simulink model "QuadcopterSimModel_INDI_Traj"  (R2018b)
settings: Solver=ode23  StartTime=0.0  StopTime=1000  FixedStep=sample_time  RelTol=1e-4  EnableMultiTasking=on
undefined symbols (not defined in the file): alt_ground, atmosphere, cycle, DiscIntNeverNeededParam, envir, fm_loiter, g, jystck, pos_ref, sigbuilder_block, traj_empty, waypoints, wind
libraries: simulink x6, ndi_lib x5, filters_lib x5, axes_transformation_lib x4, angles_lib x3, unit_conversions_lib x3, cntrl_atti_red_indi_lib x2, traj_lib x2, aerolibfltsims x2, control_allocation_lib x1, sensors_lib x1, atmosphere_lib x1
(part 3 of 3)

== matlab function QuadcopterSimModel_INDI_Traj/Controller INDI/Multicopter INDI Loiter Flight Mode/Multicopter Altitude Hold Flight Mode with INDI and reduced attitude control/control effectiveness/MATLAB Function ==
  data: ny_du_red_trim input; ny_du_dt_trim input; u_trim input; u input; G1 output; T_s input; G2 output
function [G1,G2] = controlEffectiveness2G1G2( ny_du_red_trim, ny_du_dt_trim, u_trim, u, T_s) %#codegen
[G1,G2] = controlEffectiveness2G1G2( ny_du_red_trim, ny_du_dt_trim, u_trim, u, T_s);
end

== matlab function QuadcopterSimModel_INDI_Traj/Controller INDI/Multicopter INDI Loiter Flight Mode/Multicopter Altitude Hold Flight Mode with INDI and reduced attitude control/Multicopter (Reduced) Attitude INDI Controller/reference model/MATLAB Function ==
  data: n_b_d output; n_b_d_dt output; omega_Kb input; n_b_d_dt2 output; omega_Kb_dt input; M_bg input; n_g_d input; n_g_d_dt input; n_g_d_dt2 input
function [ n_b_d, n_b_d_dt, n_b_d_dt2]   = fcn(omega_Kb, omega_Kb_dt, M_bg, n_g_d, n_g_d_dt, n_g_d_dt2 )
% https://arxiv.org/pdf/2002.07837.pdf

% time derivative of rotation matrix
M_bg_dt = dcmDerivFromOmega( M_bg', omega_Kb )';

n_b_d = M_bg*n_g_d;

n_b = single([0;0;-1]);
rho = acos( max( -1, min( 1, dot( n_b_d, n_b ) ) ) );

% eq. (7)
n_b_d_dt = -cross(omega_Kb,n_b_d) + M_bg*n_g_d_dt;

% time derivative of eq. (7)
n_b_d_dt2 = -cross(omega_Kb_dt,n_b_d) -cross(omega_Kb,n_b_d_dt) ...
    + M_bg_dt*n_g_d_dt + M_bg*n_g_d_dt2;

% manipulate desired vector if it is tilted more than 90 degrees
if n_b_d(3) > 0
    n_b_d(3) = 0;
    %n_b_d = n_b_d/(eps(n_b_d(1))+norm(n_b_d,2));
    % increase h1 and h2 up to 2 (2 for 180 degrees)
    n_b_d(1:2) = n_b_d(1:2) + 2*( n_b_d(1:2)/(eps(n_b_d(1))+norm(n_b_d(1:2),2)) - n_b_d(1:2) );
    if norm(n_b_d,2) < 0.9
        n_b_d(1) = -1;
        n_b_d = n_b_d/norm(n_b_d,2);
    end
    % sign must be flipped but it yields better results if the magnitude is
    % reduced
    n_b_d_dt = -n_b_d_dt*0.2;
    n_b_d_dt2 = -n_b_d_dt2*0.2;
end

end

== matlab function QuadcopterSimModel_INDI_Traj/Controller INDI/Multicopter INDI Loiter Flight Mode/Multicopter Altitude Hold Flight Mode with INDI and reduced attitude control/Multicopter (Reduced) Attitude INDI Controller/reference model/MATLAB Function1 ==
  data: n_b_d output; n_b_d_dt output; omega_Kb input; n_b_d_dt2 output; omega_Kb_dt input; M_bg input; n_g_d input; n_g_d_dt input; n_g_d_dt2 input
function [ n_b_d, n_b_d_dt, n_b_d_dt2]   = fcn(omega_Kb, omega_Kb_dt, M_bg, n_g_d, n_g_d_dt, n_g_d_dt2 )
% https://arxiv.org/pdf/2002.07837.pdf

% time derivative of rotation matrix
M_bg_dt = dcmDerivFromOmega( M_bg', omega_Kb )';

n_b_d = M_bg*n_g_d;

n_b = single([0;0;-1]);
rho = acos( max( -1, min( 1, dot( n_b_d, n_b ) ) ) );

% eq. (7)
n_b_d_dt = -cross(omega_Kb,n_b_d) + M_bg*n_g_d_dt;

% time derivative of eq. (7)
n_b_d_dt2 = -cross(omega_Kb_dt,n_b_d) -cross(omega_Kb,n_b_d_dt) ...
    + M_bg_dt*n_g_d_dt + M_bg*n_g_d_dt2;

% manipulate desired vector if it is tilted more than 90 degrees
if n_b_d(3) > 0
    n_b_d(3) = 0;
    %n_b_d = n_b_d/(eps(n_b_d(1))+norm(n_b_d,2));
    % increase h1 and h2 up to 2 (2 for 180 degrees)
    n_b_d(1:2) = n_b_d(1:2) + 2*( n_b_d(1:2)/(eps(n_b_d(1))+norm(n_b_d(1:2),2)) - n_b_d(1:2) );
    if norm(n_b_d,2) < 0.9
        n_b_d(1) = -1;
        n_b_d = n_b_d/norm(n_b_d,2);
    end
    % sign must be flipped but it yields better results if the magnitude is
    % reduced
    n_b_d_dt = -n_b_d_dt*0.2;
    n_b_d_dt2 = -n_b_d_dt2*0.2;
end

end

== matlab function QuadcopterSimModel_INDI_Traj/Controller INDI/Multicopter INDI Loiter Flight Mode/Waypoint Reference/waypoint Reference System/MATLAB Function1 ==
  data: M input; Psi output
function Psi = GierFromRotMatrix(M)

Theta = atan2(-M(3,1),sqrt(M(1,1).^2+ M(2,1).^2));

Psi= atan2(M(2,1)/cos(Theta),M(1,1)/cos(Theta));

== matlab function QuadcopterSimModel_INDI_Traj/Controller INDI/Multicopter INDI Loiter Flight Mode/Waypoint Reference/waypoint Reference System/MATLAB Function3 ==
  data: traj input; sec_id output; id_start input; t_start input; dist input; t output
function [sec_id,t] = trajSweepAlong(traj,id_start,t_start,dist)
[sec_id, t] = trajSweepAlong(traj,id_start,t_start,dist);

== matlab function QuadcopterSimModel_INDI_Traj/Controller INDI/Multicopter INDI Loiter Flight Mode/Multicopter Altitude Hold Flight Mode with INDI and reduced attitude control/Multicopter (Reduced) Attitude INDI Controller/reference model/lean angles 2 lean vector ==
  data: leanAngles input; n_g output
function n_g = leanAngles2leanVector( leanAngles )
n_g = leanAngles2leanVector( leanAngles );
end

== matlab function QuadcopterSimModel_INDI_Traj/Controller INDI/Multicopter INDI Loiter Flight Mode/Waypoint Reference/waypoint Reference System/MATLAB Function2 ==
  data: traj input; sec_id output; id_start input; t_start input; dist input; t output
function [sec_id,t] = trajSweepAlong(traj,id_start,t_start,dist)
[sec_id, t] = trajSweepAlong(traj,id_start,t_start,dist);

== matlab function QuadcopterSimModel_INDI_Traj/Controller INDI/Multicopter INDI Loiter Flight Mode/Horizontal NDI position (NE) controller cascade with reduced attitude (angle) command/Convert to reduced attitude pseudo control/MATLAB Function1 ==
  data: a_ref_g input; n_d_g output; g_g input
function n_d_g = fcn(a_ref_g, g_g)

n_d_g = ( a_ref_g - g_g ) / norm( a_ref_g - g_g, 2 );

end

== matlab function QuadcopterSimModel_INDI_Traj/Controller INDI/Multicopter INDI Loiter Flight Mode/Horizontal NDI position (NE) controller cascade with reduced attitude (angle) command/Convert to reduced attitude pseudo control/MATLAB Function4 ==
  data: a_ref_g input; n_d_g output; g_g input
function n_d_g = fcn(a_ref_g, g_g)

n_d_g = ( a_ref_g - g_g ) / norm( a_ref_g - g_g, 2 );

end

== matlab function QuadcopterSimModel_INDI_Traj/Controller INDI/Multicopter INDI Loiter Flight Mode/Horizontal NDI position (NE) controller cascade with reduced attitude (angle) command/Convert to reduced attitude pseudo control/MATLAB Function9 ==
  data: phi output; delta output; xyz_g_dt2 input
function [phi,delta] = fcn(xyz_g_dt2)
% function [x,y] = fcn(xyz_g_dt2)

if abs(xyz_g_dt2(3)) < 1
    if xyz_g_dt2(3) > 0
        xyz_g_dt2(3) = 1;
    else
        xyz_g_dt2(3) = -1;
    end
end

% x = atan2(xyz_g_dt2(1),-xyz_g_dt2(3));
% y = atan2(xyz_g_dt2(2),-xyz_g_dt2(3));


delta = atan2(xyz_g_dt2(2),xyz_g_dt2(1));
xy_g_dt2 = sqrt( xyz_g_dt2(1)^2 + xyz_g_dt2(2)^2 );
phi = atan2( xy_g_dt2 , -xyz_g_dt2(3) );

end

== matlab function QuadcopterSimModel_INDI_Traj/Controller INDI/Multicopter INDI Loiter Flight Mode/Waypoint Reference/waypoint Reference System/MATLAB Function ==
  data: traj input; sec_id input; acc output; vel input; g input; t input
function acc = trajSectionGetAcc(traj,sec_id,vel,g,t)
traj_sec = trajGetSection(traj,sec_id);
acc = trajSectionGetAcc(traj_sec,vel,g,t);

== matlab function QuadcopterSimModel_INDI_Traj/Controller INDI/Multicopter INDI Loiter Flight Mode/Horizontal NDI position (NE) controller cascade with reduced attitude (angle) command/Convert to reduced attitude pseudo control/MATLAB Function5 ==
  data: q_cmd input; q_e output; q_m input
function q_e = fcn(q_cmd, q_m)

q_e = quatMultiply(quatInv(q_m),q_cmd);

== matlab function QuadcopterSimModel_INDI_Traj/Controller INDI/Multicopter INDI Loiter Flight Mode/Delta attitude to stick commands/conversion to total attitude command/MATLAB Function ==
  data: u input; y output
function y = fcn(u)

y = u/norm(u,2);

== matlab function QuadcopterSimModel_INDI_Traj/Controller INDI/Multicopter INDI Loiter Flight Mode/Delta attitude to stick commands/conversion to total attitude command/MATLAB Function4 ==
  data: n_g input; phi output; delta output
function [phi,delta] = fcn(n_g)

phi = acos( max( -1, min( 1, -n_g(3) ) ) );

delta = atan2(n_g(2),n_g(1));

== matlab function QuadcopterSimModel_INDI_Traj/Controller INDI/Multicopter INDI Loiter Flight Mode/Waypoint Reference/waypoint Reference System/MATLAB Function6 ==
  data: traj input; pos output; sec_id input; t input
function pos = trajGetPos(traj, sec_id,t)
sec = trajGetSection(traj,sec_id);
pos = trajSectionGetPos(sec,t);

== matlab function QuadcopterSimModel_INDI_Traj/Controller INDI/Multicopter INDI Loiter Flight Mode/Multicopter Altitude Hold Flight Mode with INDI and reduced attitude control/Multicopter (Reduced) Attitude INDI Controller/measure/MATLAB Function1 ==
  data: q_bg input; q_red output; yaw output
function [q_red,yaw] = fcn(q_bg)
[q_red,yaw] = quatReduced(q_bg);
end

== matlab function QuadcopterSimModel_INDI_Traj/Controller INDI/Multicopter INDI Loiter Flight Mode/Delta attitude to stick commands/conversion to total attitude command/quaternion to lean angles/MATLAB Function4 ==
  data: n_g input; phi output; delta output
function [phi,delta] = fcn(n_g)

phi = acos( max( -1, min( 1, -n_g(3) ) ) );

delta = atan2(n_g(2),n_g(1));

== matlab function QuadcopterSimModel_INDI_Traj/Controller INDI/Multicopter INDI Loiter Flight Mode/Delta attitude to stick commands/conversion to total attitude command/quaternion to lean angles/quaternion to reduced attitude unit vector ==
  data: q_bg input; n_g output
function n_g = fcn( q_bg )
M_bg = quat2Dcm(q_bg);
n_g = dcm2LeanVector( M_bg );
end

== matlab function QuadcopterSimModel_INDI_Traj/Controller INDI/Multicopter INDI Loiter Flight Mode/Delta attitude to stick commands/conversion to total attitude command/total reduced attitude command (quaternion) ==
  data: q_e input; q_m input; q_cmd output
function q_cmd = fcn(q_e, q_m)

q_cmd = quatMultiply( q_m, q_e );
